simulink model "plant"  (R2025b)
settings: Solver=VariableStepAuto  StartTime=0.0  StopTime=10.0  RelTol=1e-3
libraries: eeRmsMeasurement x1, eeTotalHarmonicDistorsion x1
settings Model: Creator=Dell  LastModifiedBy=Dell

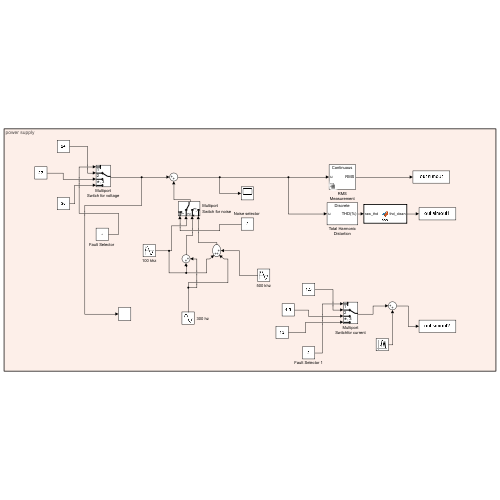
[thumbnail: Simulink's stored preview of the top-level diagram]
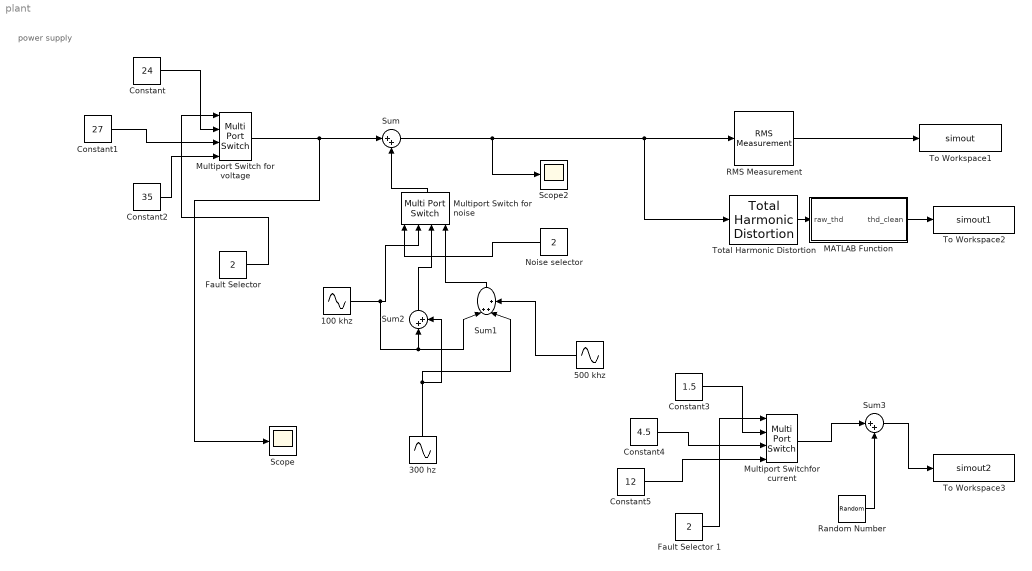
== system plant ==
  note: power supply
  100 khz : Sin  Amplitude=0.01  Frequency=628318.5  SampleTime=0
  300 hz : Sin  Amplitude=0.5  Frequency=1884955.5  SampleTime=0
  500 khz : Sin  Amplitude=2  Frequency=3141592.5  SampleTime=0
  Constant : Constant  Value=24
  Constant1 : Constant  Value=27
  Constant2 : Constant  Value=35
  Constant3 : Constant  Value=1.5
  Constant4 : Constant  Value=4.5
  Constant5 : Constant  Value=12
  "Fault Selector " : Constant  Value=2
  Fault Selector 1 : Constant  Value=2
  MATLAB Function : MATLAB Function  TreatAsAtomicUnit=on
  Multiport Switch for noise : MultiPortSwitch  SaturateOnIntegerOverflow=off  InputSameDT=off
  Multiport Switch for voltage : MultiPortSwitch  SaturateOnIntegerOverflow=off  InputSameDT=off
  Multiport Switchfor current : MultiPortSwitch  SaturateOnIntegerOverflow=off  InputSameDT=off
  "Noise selector " : Constant  Value=2
  RMS Measurement : eeRmsMeasurement/RMS Measurement  LabelModeActiveChoice=Total  F=100000  SpecifyHarmonics=off  K=[0 1 2]  Ts=0
      settings: LibrarySourceBlock=|
      | ee_sl_lib/Measurements/RMS
      | Measurement
  Random Number : RandomNumber  Variance=0.05  SampleTime=0.1
  Scope : Scope
      settings: ActiveDisplayYMinimum=-549.5374746805785  ActiveDisplayYMaximum=479.82347149424243  DataLoggingVariableName=ScopeData2  DataLoggingSaveFormat=Array
  Scope2 : Scope
      settings: ActiveDisplayYMinimum=-73.337988260736012  ActiveDisplayYMaximum=114.45534049994271  DataLoggingSaveFormat=Array
  Sum : Sum  Inputs=|++
  Sum1 : Sum  Inputs=|+++
  Sum2 : Sum  Inputs=|++
  Sum3 : Sum  Inputs=|++
  To Workspace1 : ToWorkspace  VariableName=simout  SaveFormat=Timeseries  SampleTime=-1
  To Workspace2 : ToWorkspace  VariableName=simout1  SaveFormat=Timeseries  SampleTime=-1
  To Workspace3 : ToWorkspace  VariableName=simout2  SaveFormat=Timeseries  SampleTime=-1
  Total Harmonic Distortion : eeTotalHarmonicDistorsion/Total Harmonic Distortion  f=100000  Ts=1e-6
      settings: LibrarySourceBlock=|
      | ee_sl_lib/Measurements/Total Harmonic
      | Distortion
  wires:
  Random Number/1 -> Sum3/2
  Constant1/1 -> Multiport Switch for voltage/3
  100 khz/1 -> Multiport Switch for noise/2, Sum1/1, Sum2/1
  Sum/1 -> Scope2/1, Total Harmonic Distortion/1, RMS Measurement/1
  300 hz/1 -> Sum1/2, Sum2/2
  Constant3/1 -> Multiport Switchfor current/2
  Constant/1 -> Multiport Switch for voltage/2
  Multiport Switch for voltage/1 -> Scope/1, Sum/1
  "Noise selector "/1 -> Multiport Switch for noise/1
  Constant5/1 -> Multiport Switchfor current/4
  MATLAB Function/1(thd_clean) -> To Workspace2/1
  500 khz/1 -> Sum1/3
  Fault Selector 1/1 -> Multiport Switchfor current/1
  Multiport Switch for noise/1 -> Sum/2
  Multiport Switchfor current/1 -> Sum3/1
  Total Harmonic Distortion/1 -> MATLAB Function/1(raw_thd)
  "Fault Selector "/1 -> Multiport Switch for voltage/1
  Sum2/1 -> Multiport Switch for noise/3
  RMS Measurement/1 -> To Workspace1/1
  Constant2/1 -> Multiport Switch for voltage/4
  Sum3/1 -> To Workspace3/1
  Constant4/1 -> Multiport Switchfor current/3
  Sum1/1 -> Multiport Switch for noise/4

== matlab function plant/MATLAB Function ==
  data: raw_thd input; thd_clean output
% Simple Normalization to keep Var3 between 0 and 1
function thd_clean = fcn(raw_thd)
    if raw_thd > 1
        thd_clean = 0.25; % Force a "High Fault" value for 5000+ errors
    else
        thd_clean = raw_thd;
    end
end
